simulink model "ramp_acceleration"  (R2018b)
settings: Solver=FixedStepAuto  StartTime=0.0  StopTime=10  FixedStep=0.001  RelTol=0.005
values from neighbouring files (symbols this model uses):
  A = [-b/J   K/J ... (first row only)    [motor_model.m]
  B = [0 ... (first row only)    [motor_model.m]
  C = [1   0]    [motor_model.m]
  D = 0    [motor_model.m]
settings Model: Creator=kika  LastModifiedBy=kika
settings DataIOCC: ReturnWorkspaceOutputs=on

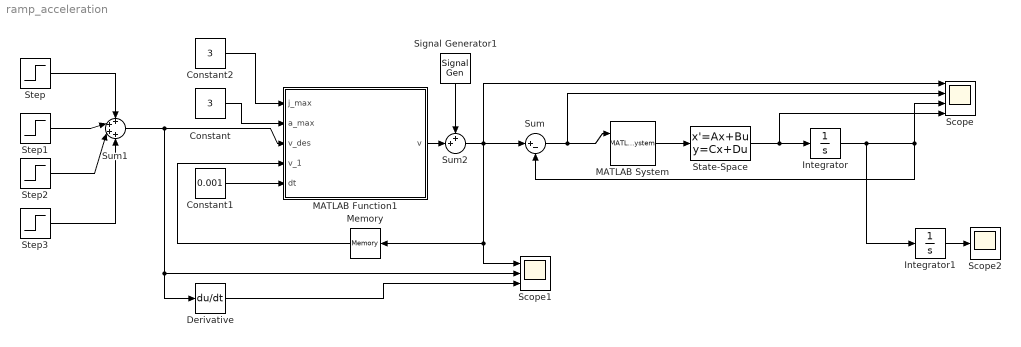
== system ramp_acceleration ==
  Constant : Constant  Value=3
  Constant1 : Constant  Value=0.001
  Constant2 : Constant  Value=3
  Derivative : Derivative
  Integrator : Integrator
  Integrator1 : Integrator
  MATLAB Function1 : MATLAB Function  TreatAsAtomicUnit=on
  MATLAB System : MATLABSystem  System=PID  dt=0.0005  kp=10  ki=0  kd=0  u_max=10  u_min=-10  ramp=false  q0=0  dq0=0  ddq0=0  q_range=[ -pi, pi ]  dq_max=pi  ddq_max=pi  dddq_max=0  antiwindup=false  kt=0  SimulateUsing=Interpreted execution
      mask Type: PID
      mask Display:
      | disp('PID');
      | port_label('input',1,'in_des');
      | port_label('input',2,'in_state');
      | port_label('output',1,'y');
  Memory : Memory
  Scope : Scope  NumInputPorts=4
  Scope1 : Scope  NumInputPorts=3
  Scope2 : Scope
  Signal Generator1 : SignalGenerator  WaveForm=random  Amplitude=0  Frequency=10  Units=rad/sec
  State-Space : StateSpace  A=A  B=B  C=C  D=D  InitialCondition=[0,0]'
  Step : Step  SampleTime=0
  Step1 : Step  Time=2  After=-1  SampleTime=0
  Step2 : Step  Time=3  After=-2  SampleTime=0
  Step3 : Step  Time=3  After=-2  SampleTime=0
  Sum : Sum  Inputs=|+-
  Sum1 : Sum  Inputs=++++
  Sum2 : Sum  Inputs=++|
  wires:
  MATLAB System/1 -> State-Space/1
  Sum/1 -> Scope/2, MATLAB System/1
  State-Space/1 -> Scope/4, Integrator/1
  Integrator/1 -> Integrator1/1, Sum/2, Scope/3
  Sum2/1 -> Sum/1, Scope/1, Memory/1, Scope1/1
  Memory/1 -> MATLAB Function1/4(v_1)
  Constant/1 -> MATLAB Function1/2(a_max)
  Step/1 -> Sum1/1
  Step1/1 -> Sum1/2
  Step2/1 -> Sum1/3
  Step3/1 -> Sum1/4
  Sum1/1 -> Scope1/2, Derivative/1, MATLAB Function1/3(v_des)
  MATLAB Function1/1(v) -> Sum2/2
  Signal Generator1/1 -> Sum2/1
  Derivative/1 -> Scope1/3
  Constant1/1 -> MATLAB Function1/5(dt)
  Integrator1/1 -> Scope2/1
  Constant2/1 -> MATLAB Function1/1(j_max)

== matlab function ramp_acceleration/MATLAB Function1 ==
  data: j_max input; a_max input; v output size=[1,1]; v_des input; v_1 input; dt input
function v = ramp_acceleration(j_max, a_max, v_des, v_1, dt)
    % if `direction`
    % `0` --velocity is constant
    % `1` -- acceleration phase
    % `-1` -- deacceleration phase
    
    direction = 0;              
    if (v_des - v_1) > eps
        direction = 1;
    elseif (v_des - v_1) < -eps
        direction = -1;
    end
    
    v = v_1 + direction * a_max * dt;
